simulink model "mce"  (Simulink 6.5)
settings: Solver=ode45  StartTime=0.0  StopTime=10.0  RelTol=1e-3
libraries: cdsFilt x334, cdsMatrix x9, cdsSwitch x7, cdsWD x7, cdsMuxMatrix x5, dac x3, cdsEpicsOut x2, cdsParameters x1
(part 10 of 18)

== system mce/Q1/M0/E/YAW ==
  In1 : Inport
  In2 : Inport  Port=2
  ADD : Subsystem
  CON : Subsystem
  SIG : Subsystem
  Out1 : Outport
  Out2 : Outport  Port=2
  Out3 : Outport  Port=3
  Out4 : Outport  Port=4
  wires:
  In1/1 -> SIG/1(In1)
  In2/1 -> CON/1(In1)
  SIG/1(Out1) -> ADD/1(In1)
  SIG/2(Out2) -> ADD/2(In2)
  SIG/3(Out3) -> ADD/3(In3)
  SIG/4(Out4) -> ADD/4(In4)
  CON/1(Out1) -> ADD/5(In17)
  CON/2(Out2) -> ADD/6(In18)
  CON/3(Out3) -> ADD/7(In19)
  CON/4(Out4) -> ADD/8(In20)
  ADD/1(Out1) -> Out1/1
  ADD/2(Out2) -> Out2/1
  ADD/3(Out3) -> Out3/1
  ADD/4(Out4) -> Out4/1

== system mce/Q1/M0/E/Z ==
  In1 : Inport
  In2 : Inport  Port=2
  ADD : Subsystem
  CON : Subsystem
  SIG : Subsystem
  Out1 : Outport
  Out2 : Outport  Port=2
  Out3 : Outport  Port=3
  Out4 : Outport  Port=4
  wires:
  In1/1 -> SIG/1(In1)
  In2/1 -> CON/1(In1)
  SIG/1(Out1) -> ADD/1(In1)
  SIG/2(Out2) -> ADD/2(In2)
  SIG/3(Out3) -> ADD/3(In3)
  SIG/4(Out4) -> ADD/4(In4)
  CON/1(Out1) -> ADD/5(In17)
  CON/2(Out2) -> ADD/6(In18)
  CON/3(Out3) -> ADD/7(In19)
  CON/4(Out4) -> ADD/8(In20)
  ADD/1(Out1) -> Out1/1
  ADD/2(Out2) -> Out2/1
  ADD/3(Out3) -> Out3/1
  ADD/4(Out4) -> Out4/1

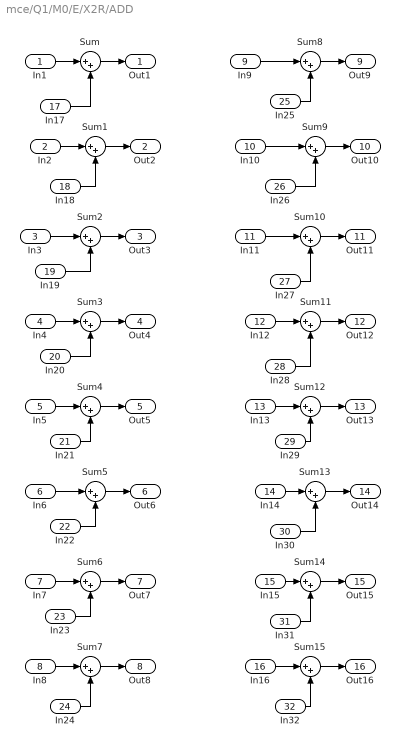
== system mce/Q1/M0/E/X2R/ADD ==
  In1 : Inport
  In2 : Inport  Port=2
  In3 : Inport  Port=3
  In4 : Inport  Port=4
  In5 : Inport  Port=5
  In6 : Inport  Port=6
  In7 : Inport  Port=7
  In8 : Inport  Port=8
  In9 : Inport  Port=9
  In10 : Inport  Port=10
  In11 : Inport  Port=11
  In12 : Inport  Port=12
  In13 : Inport  Port=13
  In14 : Inport  Port=14
  In15 : Inport  Port=15
  In16 : Inport  Port=16
  In17 : Inport  Port=17
  In18 : Inport  Port=18
  In19 : Inport  Port=19
  In20 : Inport  Port=20
  In21 : Inport  Port=21
  In22 : Inport  Port=22
  In23 : Inport  Port=23
  In24 : Inport  Port=24
  In25 : Inport  Port=25
  In26 : Inport  Port=26
  In27 : Inport  Port=27
  In28 : Inport  Port=28
  In29 : Inport  Port=29
  In30 : Inport  Port=30
  In31 : Inport  Port=31
  In32 : Inport  Port=32
  Sum{,1..15} (16 alike) : Sum  Inputs=|++
  Out1 : Outport
  Out2 : Outport  Port=2
  Out3 : Outport  Port=3
  Out4 : Outport  Port=4
  Out5 : Outport  Port=5
  Out6 : Outport  Port=6
  Out7 : Outport  Port=7
  Out8 : Outport  Port=8
  Out9 : Outport  Port=9
  Out10 : Outport  Port=10
  Out11 : Outport  Port=11
  Out12 : Outport  Port=12
  Out13 : Outport  Port=13
  Out14 : Outport  Port=14
  Out15 : Outport  Port=15
  Out16 : Outport  Port=16
  wires:
  In1/1 -> Sum/1
  Sum/1 -> Out1/1
  Sum1/1 -> Out2/1
  Sum2/1 -> Out3/1
  Sum3/1 -> Out4/1
  Sum4/1 -> Out5/1
  Sum5/1 -> Out6/1
  Sum6/1 -> Out7/1
  Sum7/1 -> Out8/1
  Sum8/1 -> Out9/1
  Sum9/1 -> Out10/1
  Sum10/1 -> Out11/1
  Sum11/1 -> Out12/1
  Sum12/1 -> Out13/1
  Sum13/1 -> Out14/1
  Sum14/1 -> Out15/1
  Sum15/1 -> Out16/1
  In17/1 -> Sum/2
  In2/1 -> Sum1/1
  In3/1 -> Sum2/1
  In4/1 -> Sum3/1
  In5/1 -> Sum4/1
  In19/1 -> Sum2/2
  In20/1 -> Sum3/2
  In21/1 -> Sum4/2
  In6/1 -> Sum5/1
  In22/1 -> Sum5/2
  In7/1 -> Sum6/1
  In23/1 -> Sum6/2
  In8/1 -> Sum7/1
  In24/1 -> Sum7/2
  In9/1 -> Sum8/1
  In25/1 -> Sum8/2
  In10/1 -> Sum9/1
  In26/1 -> Sum9/2
  In11/1 -> Sum10/1
  In27/1 -> Sum10/2
  In12/1 -> Sum11/1
  In28/1 -> Sum11/2
  In13/1 -> Sum12/1
  In29/1 -> Sum12/2
  In14/1 -> Sum13/1
  In30/1 -> Sum13/2
  In15/1 -> Sum14/1
  In31/1 -> Sum14/2
  In16/1 -> Sum15/1
  In32/1 -> Sum15/2
  In18/1 -> Sum1/2

== system mce/Q1/M0/E/X2R/CON ==
  In1 : Inport
  In2 : Inport  Port=2
  In3 : Inport  Port=3
  In4 : Inport  Port=4
  ADD : Subsystem
  ADD1 : Subsystem
  ADD3 : Subsystem
  P : Subsystem
  R : Subsystem
  X : Subsystem
  Y : Subsystem
  Out1 : Outport
  Out2 : Outport  Port=2
  Out3 : Outport  Port=3
  Out4 : Outport  Port=4
  Out5 : Outport  Port=5
  Out6 : Outport  Port=6
  Out7 : Outport  Port=7
  Out8 : Outport  Port=8
  Out9 : Outport  Port=9
  Out10 : Outport  Port=10
  Out11 : Outport  Port=11
  Out12 : Outport  Port=12
  Out13 : Outport  Port=13
  Out14 : Outport  Port=14
  Out15 : Outport  Port=15
  Out16 : Outport  Port=16
  wires:
  In1/1 -> X/1(In1)
  In2/1 -> Y/1(In1)
  X/1(Out1) -> ADD/1(In1)
  X/2(Out2) -> ADD/2(In2)
  X/3(Out3) -> ADD/3(In3)
  X/4(Out4) -> ADD/4(In4)
  X/5(Out5) -> ADD/5(In5)
  X/6(Out6) -> ADD/6(In6)
  X/7(Out7) -> ADD/7(In7)
  X/8(Out8) -> ADD/8(In8)
  X/9(Out9) -> ADD/9(In9)
  X/10(Out10) -> ADD/10(In10)
  X/11(Out11) -> ADD/11(In11)
  X/12(Out12) -> ADD/12(In12)
  X/13(Out13) -> ADD/13(In13)
  X/14(Out14) -> ADD/14(In14)
  X/15(Out15) -> ADD/15(In15)
  X/16(Out16) -> ADD/16(In16)
  In3/1 -> P/1(In1)
  In4/1 -> R/1(In1)
  ADD/1(Out1) -> ADD3/1(In1)
  ADD/2(Out2) -> ADD3/2(In2)
  ADD/3(Out3) -> ADD3/3(In3)
  ADD/4(Out4) -> ADD3/4(In4)
  ADD/5(Out5) -> ADD3/5(In5)
  ADD/6(Out6) -> ADD3/6(In6)
  ADD/7(Out7) -> ADD3/7(In7)
  ADD/8(Out8) -> ADD3/8(In8)
  ADD/9(Out9) -> ADD3/9(In9)
  ADD/10(Out10) -> ADD3/10(In10)
  ADD/11(Out11) -> ADD3/11(In11)
  ADD/12(Out12) -> ADD3/12(In12)
  ADD/13(Out13) -> ADD3/13(In13)
  ADD/14(Out14) -> ADD3/14(In14)
  ADD/15(Out15) -> ADD3/15(In15)
  ADD/16(Out16) -> ADD3/16(In16)
  ADD1/1(Out1) -> ADD3/17(In17)
  ADD1/2(Out2) -> ADD3/18(In18)
  ADD1/3(Out3) -> ADD3/19(In19)
  ADD1/4(Out4) -> ADD3/20(In20)
  ADD1/5(Out5) -> ADD3/21(In21)
  ADD1/6(Out6) -> ADD3/22(In22)
  ADD1/7(Out7) -> ADD3/23(In23)
  ADD1/8(Out8) -> ADD3/24(In24)
  ADD1/9(Out9) -> ADD3/25(In25)
  ADD1/10(Out10) -> ADD3/26(In26)
  ADD1/11(Out11) -> ADD3/27(In27)
  ADD1/12(Out12) -> ADD3/28(In28)
  ADD1/13(Out13) -> ADD3/29(In29)
  ADD1/14(Out14) -> ADD3/30(In30)
  ADD1/15(Out15) -> ADD3/31(In31)
  ADD1/16(Out16) -> ADD3/32(In32)
  ADD3/1(Out1) -> Out1/1
  ADD3/2(Out2) -> Out2/1
  ADD3/3(Out3) -> Out3/1
  ADD3/4(Out4) -> Out4/1
  ADD3/5(Out5) -> Out5/1
  ADD3/6(Out6) -> Out6/1
  ADD3/7(Out7) -> Out7/1
  ADD3/8(Out8) -> Out8/1
  ADD3/9(Out9) -> Out9/1
  ADD3/10(Out10) -> Out10/1
  ADD3/11(Out11) -> Out11/1
  ADD3/12(Out12) -> Out12/1
  ADD3/13(Out13) -> Out13/1
  ADD3/14(Out14) -> Out14/1
  ADD3/15(Out15) -> Out15/1
  ADD3/16(Out16) -> Out16/1
  Y/1(Out1) -> ADD/17(In17)
  Y/2(Out2) -> ADD/18(In18)
  Y/3(Out3) -> ADD/19(In19)
  Y/4(Out4) -> ADD/20(In20)
  Y/5(Out5) -> ADD/21(In21)
  Y/6(Out6) -> ADD/22(In22)
  Y/7(Out7) -> ADD/23(In23)
  Y/8(Out8) -> ADD/24(In24)
  Y/9(Out9) -> ADD/25(In25)
  Y/10(Out10) -> ADD/26(In26)
  Y/11(Out11) -> ADD/27(In27)
  Y/12(Out12) -> ADD/28(In28)
  Y/13(Out13) -> ADD/29(In29)
  Y/14(Out14) -> ADD/30(In30)
  Y/15(Out15) -> ADD/31(In31)
  Y/16(Out16) -> ADD/32(In32)
  P/1(Out1) -> ADD1/1(In1)
  P/2(Out2) -> ADD1/2(In2)
  P/3(Out3) -> ADD1/3(In3)
  P/4(Out4) -> ADD1/4(In4)
  P/5(Out5) -> ADD1/5(In5)
  P/6(Out6) -> ADD1/6(In6)
  P/7(Out7) -> ADD1/7(In7)
  P/8(Out8) -> ADD1/8(In8)
  P/9(Out9) -> ADD1/9(In9)
  P/10(Out10) -> ADD1/10(In10)
  P/11(Out11) -> ADD1/11(In11)
  P/12(Out12) -> ADD1/12(In12)
  P/13(Out13) -> ADD1/13(In13)
  P/14(Out14) -> ADD1/14(In14)
  P/15(Out15) -> ADD1/15(In15)
  P/16(Out16) -> ADD1/16(In16)
  R/1(Out1) -> ADD1/17(In17)
  R/2(Out2) -> ADD1/18(In18)
  R/3(Out3) -> ADD1/19(In19)
  R/4(Out4) -> ADD1/20(In20)
  R/5(Out5) -> ADD1/21(In21)
  R/6(Out6) -> ADD1/22(In22)
  R/7(Out7) -> ADD1/23(In23)
  R/8(Out8) -> ADD1/24(In24)
  R/9(Out9) -> ADD1/25(In25)
  R/10(Out10) -> ADD1/26(In26)
  R/11(Out11) -> ADD1/27(In27)
  R/12(Out12) -> ADD1/28(In28)
  R/13(Out13) -> ADD1/29(In29)
  R/14(Out14) -> ADD1/30(In30)
  R/15(Out15) -> ADD1/31(In31)
  R/16(Out16) -> ADD1/32(In32)

== system mce/Q1/M0/E/X2R/SIG ==
  In1 : Inport
  In2 : Inport  Port=2
  In3 : Inport  Port=3
  In4 : Inport  Port=4
  ADD : Subsystem
  ADD1 : Subsystem
  ADD3 : Subsystem
  P : Subsystem
  R : Subsystem
  X : Subsystem
  Y : Subsystem
  Out1 : Outport
  Out2 : Outport  Port=2
  Out3 : Outport  Port=3
  Out4 : Outport  Port=4
  Out5 : Outport  Port=5
  Out6 : Outport  Port=6
  Out7 : Outport  Port=7
  Out8 : Outport  Port=8
  Out9 : Outport  Port=9
  Out10 : Outport  Port=10
  Out11 : Outport  Port=11
  Out12 : Outport  Port=12
  Out13 : Outport  Port=13
  Out14 : Outport  Port=14
  Out15 : Outport  Port=15
  Out16 : Outport  Port=16
  wires:
  In1/1 -> X/1(In1)
  In2/1 -> Y/1(In1)
  X/1(Out1) -> ADD/1(In1)
  X/2(Out2) -> ADD/2(In2)
  X/3(Out3) -> ADD/3(In3)
  X/4(Out4) -> ADD/4(In4)
  X/5(Out5) -> ADD/5(In5)
  X/6(Out6) -> ADD/6(In6)
  X/7(Out7) -> ADD/7(In7)
  X/8(Out8) -> ADD/8(In8)
  X/9(Out9) -> ADD/9(In9)
  X/10(Out10) -> ADD/10(In10)
  X/11(Out11) -> ADD/11(In11)
  X/12(Out12) -> ADD/12(In12)
  X/13(Out13) -> ADD/13(In13)
  X/14(Out14) -> ADD/14(In14)
  X/15(Out15) -> ADD/15(In15)
  X/16(Out16) -> ADD/16(In16)
  In3/1 -> P/1(In1)
  In4/1 -> R/1(In1)
  ADD/1(Out1) -> ADD3/1(In1)
  ADD/2(Out2) -> ADD3/2(In2)
  ADD/3(Out3) -> ADD3/3(In3)
  ADD/4(Out4) -> ADD3/4(In4)
  ADD/5(Out5) -> ADD3/5(In5)
  ADD/6(Out6) -> ADD3/6(In6)
  ADD/7(Out7) -> ADD3/7(In7)
  ADD/8(Out8) -> ADD3/8(In8)
  ADD/9(Out9) -> ADD3/9(In9)
  ADD/10(Out10) -> ADD3/10(In10)
  ADD/11(Out11) -> ADD3/11(In11)
  ADD/12(Out12) -> ADD3/12(In12)
  ADD/13(Out13) -> ADD3/13(In13)
  ADD/14(Out14) -> ADD3/14(In14)
  ADD/15(Out15) -> ADD3/15(In15)
  ADD/16(Out16) -> ADD3/16(In16)
  ADD1/1(Out1) -> ADD3/17(In17)
  ADD1/2(Out2) -> ADD3/18(In18)
  ADD1/3(Out3) -> ADD3/19(In19)
  ADD1/4(Out4) -> ADD3/20(In20)
  ADD1/5(Out5) -> ADD3/21(In21)
  ADD1/6(Out6) -> ADD3/22(In22)
  ADD1/7(Out7) -> ADD3/23(In23)
  ADD1/8(Out8) -> ADD3/24(In24)
  ADD1/9(Out9) -> ADD3/25(In25)
  ADD1/10(Out10) -> ADD3/26(In26)
  ADD1/11(Out11) -> ADD3/27(In27)
  ADD1/12(Out12) -> ADD3/28(In28)
  ADD1/13(Out13) -> ADD3/29(In29)
  ADD1/14(Out14) -> ADD3/30(In30)
  ADD1/15(Out15) -> ADD3/31(In31)
  ADD1/16(Out16) -> ADD3/32(In32)
  ADD3/1(Out1) -> Out1/1
  ADD3/2(Out2) -> Out2/1
  ADD3/3(Out3) -> Out3/1
  ADD3/4(Out4) -> Out4/1
  ADD3/5(Out5) -> Out5/1
  ADD3/6(Out6) -> Out6/1
  ADD3/7(Out7) -> Out7/1
  ADD3/8(Out8) -> Out8/1
  ADD3/9(Out9) -> Out9/1
  ADD3/10(Out10) -> Out10/1
  ADD3/11(Out11) -> Out11/1
  ADD3/12(Out12) -> Out12/1
  ADD3/13(Out13) -> Out13/1
  ADD3/14(Out14) -> Out14/1
  ADD3/15(Out15) -> Out15/1
  ADD3/16(Out16) -> Out16/1
  Y/1(Out1) -> ADD/17(In17)
  Y/2(Out2) -> ADD/18(In18)
  Y/3(Out3) -> ADD/19(In19)
  Y/4(Out4) -> ADD/20(In20)
  Y/5(Out5) -> ADD/21(In21)
  Y/6(Out6) -> ADD/22(In22)
  Y/7(Out7) -> ADD/23(In23)
  Y/8(Out8) -> ADD/24(In24)
  Y/9(Out9) -> ADD/25(In25)
  Y/10(Out10) -> ADD/26(In26)
  Y/11(Out11) -> ADD/27(In27)
  Y/12(Out12) -> ADD/28(In28)
  Y/13(Out13) -> ADD/29(In29)
  Y/14(Out14) -> ADD/30(In30)
  Y/15(Out15) -> ADD/31(In31)
  Y/16(Out16) -> ADD/32(In32)
  P/1(Out1) -> ADD1/1(In1)
  P/2(Out2) -> ADD1/2(In2)
  P/3(Out3) -> ADD1/3(In3)
  P/4(Out4) -> ADD1/4(In4)
  P/5(Out5) -> ADD1/5(In5)
  P/6(Out6) -> ADD1/6(In6)
  P/7(Out7) -> ADD1/7(In7)
  P/8(Out8) -> ADD1/8(In8)
  P/9(Out9) -> ADD1/9(In9)
  P/10(Out10) -> ADD1/10(In10)
  P/11(Out11) -> ADD1/11(In11)
  P/12(Out12) -> ADD1/12(In12)
  P/13(Out13) -> ADD1/13(In13)
  P/14(Out14) -> ADD1/14(In14)
  P/15(Out15) -> ADD1/15(In15)
  P/16(Out16) -> ADD1/16(In16)
  R/1(Out1) -> ADD1/17(In17)
  R/2(Out2) -> ADD1/18(In18)
  R/3(Out3) -> ADD1/19(In19)
  R/4(Out4) -> ADD1/20(In20)
  R/5(Out5) -> ADD1/21(In21)
  R/6(Out6) -> ADD1/22(In22)
  R/7(Out7) -> ADD1/23(In23)
  R/8(Out8) -> ADD1/24(In24)
  R/9(Out9) -> ADD1/25(In25)
  R/10(Out10) -> ADD1/26(In26)
  R/11(Out11) -> ADD1/27(In27)
  R/12(Out12) -> ADD1/28(In28)
  R/13(Out13) -> ADD1/29(In29)
  R/14(Out14) -> ADD1/30(In30)
  R/15(Out15) -> ADD1/31(In31)
  R/16(Out16) -> ADD1/32(In32)

== system mce/Q1/M0/E/YAW/ADD ==
  In1 : Inport
  In2 : Inport  Port=2
  In3 : Inport  Port=3
  In4 : Inport  Port=4
  In17 : Inport  Port=5
  In18 : Inport  Port=6
  In19 : Inport  Port=7
  In20 : Inport  Port=8
  Sum{,1..3} (4 alike) : Sum  Inputs=|++
  Out1 : Outport
  Out2 : Outport  Port=2
  Out3 : Outport  Port=3
  Out4 : Outport  Port=4
  wires:
  In1/1 -> Sum/1
  Sum/1 -> Out1/1
  Sum1/1 -> Out2/1
  Sum2/1 -> Out3/1
  Sum3/1 -> Out4/1
  In17/1 -> Sum/2
  In2/1 -> Sum1/1
  In3/1 -> Sum2/1
  In4/1 -> Sum3/1
  In19/1 -> Sum2/2
  In20/1 -> Sum3/2
  In18/1 -> Sum1/2

== system mce/Q1/M0/E/YAW/CON ==
  In1 : Inport
  M1 : cdsFilt/Subsystem  Tag=cdsFilt  Description=|  SystemSampleTime=-1
      | Purpose:                                                                                                                                                                                                                                  
      | Standard CDS IIR filter module.                                                                                                                                                                                                           
      |                                                                                                                                                                                                                                           
      | Operation:                                                                                                                                                                                                                                
      | Consists of 10 second order section IIR filters, plus a ramped gain stage. In FE code, also provides pre-defined test points and excitation channel inputs. The filter coefficients are defined in the LIGO system using the 'foton' tool.
      |                                                                                                                                                                                                                                           
      | Usage:                                                                                                                                                                                                                                    
      | Name the part with the desired filter module name.
      settings: AttributesFormatString=%<Tag>
  M2 : cdsFilt/Subsystem  Tag=cdsFilt  Description=|  SystemSampleTime=-1
      | Purpose:                                                                                                                                                                                                                                  
      | Standard CDS IIR filter module.                                                                                                                                                                                                           
      |                                                                                                                                                                                                                                           
      | Operation:                                                                                                                                                                                                                                
      | Consists of 10 second order section IIR filters, plus a ramped gain stage. In FE code, also provides pre-defined test points and excitation channel inputs. The filter coefficients are defined in the LIGO system using the 'foton' tool.
      |                                                                                                                                                                                                                                           
      | Usage:                                                                                                                                                                                                                                    
      | Name the part with the desired filter module name.
      settings: AttributesFormatString=%<Tag>
  M3 : cdsFilt/Subsystem  Tag=cdsFilt  Description=|  SystemSampleTime=-1
      | Purpose:                                                                                                                                                                                                                                  
      | Standard CDS IIR filter module.                                                                                                                                                                                                           
      |                                                                                                                                                                                                                                           
      | Operation:                                                                                                                                                                                                                                
      | Consists of 10 second order section IIR filters, plus a ramped gain stage. In FE code, also provides pre-defined test points and excitation channel inputs. The filter coefficients are defined in the LIGO system using the 'foton' tool.
      |                                                                                                                                                                                                                                           
      | Usage:                                                                                                                                                                                                                                    
      | Name the part with the desired filter module name.
      settings: AttributesFormatString=%<Tag>
  M4 : cdsFilt/Subsystem  Tag=cdsFilt  Description=|  SystemSampleTime=-1
      | Purpose:                                                                                                                                                                                                                                  
      | Standard CDS IIR filter module.                                                                                                                                                                                                           
      |                                                                                                                                                                                                                                           
      | Operation:                                                                                                                                                                                                                                
      | Consists of 10 second order section IIR filters, plus a ramped gain stage. In FE code, also provides pre-defined test points and excitation channel inputs. The filter coefficients are defined in the LIGO system using the 'foton' tool.
      |                                                                                                                                                                                                                                           
      | Usage:                                                                                                                                                                                                                                    
      | Name the part with the desired filter module name.
      settings: AttributesFormatString=%<Tag>
  Out1 : Outport
  Out2 : Outport  Port=2
  Out3 : Outport  Port=3
  Out4 : Outport  Port=4
  wires:
  M1/1 -> Out1/1
  M2/1 -> Out2/1
  M3/1 -> Out3/1
  M4/1 -> Out4/1
  In1/1 -> M1/1, M2/1, M3/1, M4/1

== system mce/Q1/M0/E/YAW/SIG ==
  In1 : Inport
  M1 : cdsFilt/Subsystem  Tag=cdsFilt  Description=|  SystemSampleTime=-1
      | Purpose:                                                                                                                                                                                                                                  
      | Standard CDS IIR filter module.                                                                                                                                                                                                           
      |                                                                                                                                                                                                                                           
      | Operation:                                                                                                                                                                                                                                
      | Consists of 10 second order section IIR filters, plus a ramped gain stage. In FE code, also provides pre-defined test points and excitation channel inputs. The filter coefficients are defined in the LIGO system using the 'foton' tool.
      |                                                                                                                                                                                                                                           
      | Usage:                                                                                                                                                                                                                                    
      | Name the part with the desired filter module name.
      settings: AttributesFormatString=%<Tag>
  M2 : cdsFilt/Subsystem  Tag=cdsFilt  Description=|  SystemSampleTime=-1
      | Purpose:                                                                                                                                                                                                                                  
      | Standard CDS IIR filter module.                                                                                                                                                                                                           
      |                                                                                                                                                                                                                                           
      | Operation:                                                                                                                                                                                                                                
      | Consists of 10 second order section IIR filters, plus a ramped gain stage. In FE code, also provides pre-defined test points and excitation channel inputs. The filter coefficients are defined in the LIGO system using the 'foton' tool.
      |                                                                                                                                                                                                                                           
      | Usage:                                                                                                                                                                                                                                    
      | Name the part with the desired filter module name.
      settings: AttributesFormatString=%<Tag>
  M3 : cdsFilt/Subsystem  Tag=cdsFilt  Description=|  SystemSampleTime=-1
      | Purpose:                                                                                                                                                                                                                                  
      | Standard CDS IIR filter module.                                                                                                                                                                                                           
      |                                                                                                                                                                                                                                           
      | Operation:                                                                                                                                                                                                                                
      | Consists of 10 second order section IIR filters, plus a ramped gain stage. In FE code, also provides pre-defined test points and excitation channel inputs. The filter coefficients are defined in the LIGO system using the 'foton' tool.
      |                                                                                                                                                                                                                                           
      | Usage:                                                                                                                                                                                                                                    
      | Name the part with the desired filter module name.
      settings: AttributesFormatString=%<Tag>
  M4 : cdsFilt/Subsystem  Tag=cdsFilt  Description=|  SystemSampleTime=-1
      | Purpose:                                                                                                                                                                                                                                  
      | Standard CDS IIR filter module.                                                                                                                                                                                                           
      |                                                                                                                                                                                                                                           
      | Operation:                                                                                                                                                                                                                                
      | Consists of 10 second order section IIR filters, plus a ramped gain stage. In FE code, also provides pre-defined test points and excitation channel inputs. The filter coefficients are defined in the LIGO system using the 'foton' tool.
      |                                                                                                                                                                                                                                           
      | Usage:                                                                                                                                                                                                                                    
      | Name the part with the desired filter module name.
      settings: AttributesFormatString=%<Tag>
  Out1 : Outport
  Out2 : Outport  Port=2
  Out3 : Outport  Port=3
  Out4 : Outport  Port=4
  wires:
  M1/1 -> Out1/1
  M2/1 -> Out2/1
  M3/1 -> Out3/1
  M4/1 -> Out4/1
  In1/1 -> M2/1, M3/1, M4/1, M1/1

== system mce/Q1/M0/E/Z/ADD ==
  In1 : Inport
  In2 : Inport  Port=2
  In3 : Inport  Port=3
  In4 : Inport  Port=4
  In17 : Inport  Port=5
  In18 : Inport  Port=6
  In19 : Inport  Port=7
  In20 : Inport  Port=8
  Sum{,1..3} (4 alike) : Sum  Inputs=|++
  Out1 : Outport
  Out2 : Outport  Port=2
  Out3 : Outport  Port=3
  Out4 : Outport  Port=4
  wires:
  In1/1 -> Sum/1
  Sum/1 -> Out1/1
  Sum1/1 -> Out2/1
  Sum2/1 -> Out3/1
  Sum3/1 -> Out4/1
  In17/1 -> Sum/2
  In2/1 -> Sum1/1
  In3/1 -> Sum2/1
  In4/1 -> Sum3/1
  In19/1 -> Sum2/2
  In20/1 -> Sum3/2
  In18/1 -> Sum1/2

== system mce/Q1/M0/E/Z/CON ==
  In1 : Inport
  M1 : cdsFilt/Subsystem  Tag=cdsFilt  Description=|  SystemSampleTime=-1
      | Purpose:                                                                                                                                                                                                                                  
      | Standard CDS IIR filter module.                                                                                                                                                                                                           
      |                                                                                                                                                                                                                                           
      | Operation:                                                                                                                                                                                                                                
      | Consists of 10 second order section IIR filters, plus a ramped gain stage. In FE code, also provides pre-defined test points and excitation channel inputs. The filter coefficients are defined in the LIGO system using the 'foton' tool.
      |                                                                                                                                                                                                                                           
      | Usage:                                                                                                                                                                                                                                    
      | Name the part with the desired filter module name.
      settings: AttributesFormatString=%<Tag>
  M2 : cdsFilt/Subsystem  Tag=cdsFilt  Description=|  SystemSampleTime=-1
      | Purpose:                                                                                                                                                                                                                                  
      | Standard CDS IIR filter module.                                                                                                                                                                                                           
      |                                                                                                                                                                                                                                           
      | Operation:                                                                                                                                                                                                                                
      | Consists of 10 second order section IIR filters, plus a ramped gain stage. In FE code, also provides pre-defined test points and excitation channel inputs. The filter coefficients are defined in the LIGO system using the 'foton' tool.
      |                                                                                                                                                                                                                                           
      | Usage:                                                                                                                                                                                                                                    
      | Name the part with the desired filter module name.
      settings: AttributesFormatString=%<Tag>
  M3 : cdsFilt/Subsystem  Tag=cdsFilt  Description=|  SystemSampleTime=-1
      | Purpose:                                                                                                                                                                                                                                  
      | Standard CDS IIR filter module.                                                                                                                                                                                                           
      |                                                                                                                                                                                                                                           
      | Operation:                                                                                                                                                                                                                                
      | Consists of 10 second order section IIR filters, plus a ramped gain stage. In FE code, also provides pre-defined test points and excitation channel inputs. The filter coefficients are defined in the LIGO system using the 'foton' tool.
      |                                                                                                                                                                                                                                           
      | Usage:                                                                                                                                                                                                                                    
      | Name the part with the desired filter module name.
      settings: AttributesFormatString=%<Tag>
  M4 : cdsFilt/Subsystem  Tag=cdsFilt  Description=|  SystemSampleTime=-1
      | Purpose:                                                                                                                                                                                                                                  
      | Standard CDS IIR filter module.                                                                                                                                                                                                           
      |                                                                                                                                                                                                                                           
      | Operation:                                                                                                                                                                                                                                
      | Consists of 10 second order section IIR filters, plus a ramped gain stage. In FE code, also provides pre-defined test points and excitation channel inputs. The filter coefficients are defined in the LIGO system using the 'foton' tool.
      |                                                                                                                                                                                                                                           
      | Usage:                                                                                                                                                                                                                                    
      | Name the part with the desired filter module name.
      settings: AttributesFormatString=%<Tag>
  Out1 : Outport
  Out2 : Outport  Port=2
  Out3 : Outport  Port=3
  Out4 : Outport  Port=4
  wires:
  M1/1 -> Out1/1
  M2/1 -> Out2/1
  M3/1 -> Out3/1
  M4/1 -> Out4/1
  In1/1 -> M1/1, M2/1, M3/1, M4/1

== system mce/Q1/M0/E/Z/SIG ==
  In1 : Inport
  M1 : cdsFilt/Subsystem  Tag=cdsFilt  Description=|  SystemSampleTime=-1
      | Purpose:                                                                                                                                                                                                                                  
      | Standard CDS IIR filter module.                                                                                                                                                                                                           
      |                                                                                                                                                                                                                                           
      | Operation:                                                                                                                                                                                                                                
      | Consists of 10 second order section IIR filters, plus a ramped gain stage. In FE code, also provides pre-defined test points and excitation channel inputs. The filter coefficients are defined in the LIGO system using the 'foton' tool.
      |                                                                                                                                                                                                                                           
      | Usage:                                                                                                                                                                                                                                    
      | Name the part with the desired filter module name.
      settings: AttributesFormatString=%<Tag>
  M2 : cdsFilt/Subsystem  Tag=cdsFilt  Description=|  SystemSampleTime=-1
      | Purpose:                                                                                                                                                                                                                                  
      | Standard CDS IIR filter module.                                                                                                                                                                                                           
      |                                                                                                                                                                                                                                           
      | Operation:                                                                                                                                                                                                                                
      | Consists of 10 second order section IIR filters, plus a ramped gain stage. In FE code, also provides pre-defined test points and excitation channel inputs. The filter coefficients are defined in the LIGO system using the 'foton' tool.
      |                                                                                                                                                                                                                                           
      | Usage:                                                                                                                                                                                                                                    
      | Name the part with the desired filter module name.
      settings: AttributesFormatString=%<Tag>
  M3 : cdsFilt/Subsystem  Tag=cdsFilt  Description=|  SystemSampleTime=-1
      | Purpose:                                                                                                                                                                                                                                  
      | Standard CDS IIR filter module.                                                                                                                                                                                                           
      |                                                                                                                                                                                                                                           
      | Operation:                                                                                                                                                                                                                                
      | Consists of 10 second order section IIR filters, plus a ramped gain stage. In FE code, also provides pre-defined test points and excitation channel inputs. The filter coefficients are defined in the LIGO system using the 'foton' tool.
      |                                                                                                                                                                                                                                           
      | Usage:                                                                                                                                                                                                                                    
      | Name the part with the desired filter module name.
      settings: AttributesFormatString=%<Tag>
  M4 : cdsFilt/Subsystem  Tag=cdsFilt  Description=|  SystemSampleTime=-1
      | Purpose:                                                                                                                                                                                                                                  
      | Standard CDS IIR filter module.                                                                                                                                                                                                           
      |                                                                                                                                                                                                                                           
      | Operation:                                                                                                                                                                                                                                
      | Consists of 10 second order section IIR filters, plus a ramped gain stage. In FE code, also provides pre-defined test points and excitation channel inputs. The filter coefficients are defined in the LIGO system using the 'foton' tool.
      |                                                                                                                                                                                                                                           
      | Usage:                                                                                                                                                                                                                                    
      | Name the part with the desired filter module name.
      settings: AttributesFormatString=%<Tag>
  Out1 : Outport
  Out2 : Outport  Port=2
  Out3 : Outport  Port=3
  Out4 : Outport  Port=4
  wires:
  M1/1 -> Out1/1
  M2/1 -> Out2/1
  M3/1 -> Out3/1
  M4/1 -> Out4/1
  In1/1 -> M2/1, M3/1, M4/1, M1/1

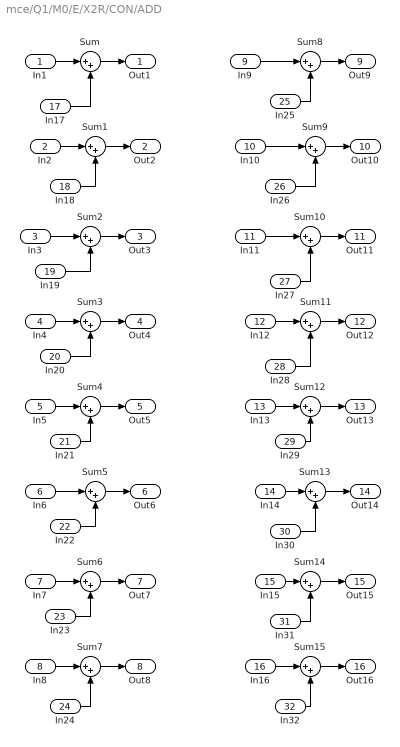
== system mce/Q1/M0/E/X2R/CON/ADD ==
  In1 : Inport
  In2 : Inport  Port=2
  In3 : Inport  Port=3
  In4 : Inport  Port=4
  In5 : Inport  Port=5
  In6 : Inport  Port=6
  In7 : Inport  Port=7
  In8 : Inport  Port=8
  In9 : Inport  Port=9
  In10 : Inport  Port=10
  In11 : Inport  Port=11
  In12 : Inport  Port=12
  In13 : Inport  Port=13
  In14 : Inport  Port=14
  In15 : Inport  Port=15
  In16 : Inport  Port=16
  In17 : Inport  Port=17
  In18 : Inport  Port=18
  In19 : Inport  Port=19
  In20 : Inport  Port=20
  In21 : Inport  Port=21
  In22 : Inport  Port=22
  In23 : Inport  Port=23
  In24 : Inport  Port=24
  In25 : Inport  Port=25
  In26 : Inport  Port=26
  In27 : Inport  Port=27
  In28 : Inport  Port=28
  In29 : Inport  Port=29
  In30 : Inport  Port=30
  In31 : Inport  Port=31
  In32 : Inport  Port=32
  Sum{,1..15} (16 alike) : Sum  Inputs=|++
  Out1 : Outport
  Out2 : Outport  Port=2
  Out3 : Outport  Port=3
  Out4 : Outport  Port=4
  Out5 : Outport  Port=5
  Out6 : Outport  Port=6
  Out7 : Outport  Port=7
  Out8 : Outport  Port=8
  Out9 : Outport  Port=9
  Out10 : Outport  Port=10
  Out11 : Outport  Port=11
  Out12 : Outport  Port=12
  Out13 : Outport  Port=13
  Out14 : Outport  Port=14
  Out15 : Outport  Port=15
  Out16 : Outport  Port=16
  wires:
  In1/1 -> Sum/1
  Sum/1 -> Out1/1
  Sum1/1 -> Out2/1
  Sum2/1 -> Out3/1
  Sum3/1 -> Out4/1
  Sum4/1 -> Out5/1
  Sum5/1 -> Out6/1
  Sum6/1 -> Out7/1
  Sum7/1 -> Out8/1
  Sum8/1 -> Out9/1
  Sum9/1 -> Out10/1
  Sum10/1 -> Out11/1
  Sum11/1 -> Out12/1
  Sum12/1 -> Out13/1
  Sum13/1 -> Out14/1
  Sum14/1 -> Out15/1
  Sum15/1 -> Out16/1
  In17/1 -> Sum/2
  In2/1 -> Sum1/1
  In3/1 -> Sum2/1
  In4/1 -> Sum3/1
  In5/1 -> Sum4/1
  In19/1 -> Sum2/2
  In20/1 -> Sum3/2
  In21/1 -> Sum4/2
  In6/1 -> Sum5/1
  In22/1 -> Sum5/2
  In7/1 -> Sum6/1
  In23/1 -> Sum6/2
  In8/1 -> Sum7/1
  In24/1 -> Sum7/2
  In9/1 -> Sum8/1
  In25/1 -> Sum8/2
  In10/1 -> Sum9/1
  In26/1 -> Sum9/2
  In11/1 -> Sum10/1
  In27/1 -> Sum10/2
  In12/1 -> Sum11/1
  In28/1 -> Sum11/2
  In13/1 -> Sum12/1
  In29/1 -> Sum12/2
  In14/1 -> Sum13/1
  In30/1 -> Sum13/2
  In15/1 -> Sum14/1
  In31/1 -> Sum14/2
  In16/1 -> Sum15/1
  In32/1 -> Sum15/2
  In18/1 -> Sum1/2

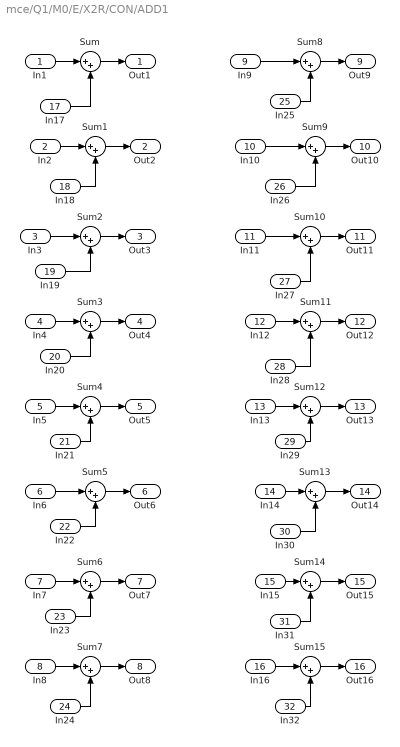
== system mce/Q1/M0/E/X2R/CON/ADD1 ==
  In1 : Inport
  In2 : Inport  Port=2
  In3 : Inport  Port=3
  In4 : Inport  Port=4
  In5 : Inport  Port=5
  In6 : Inport  Port=6
  In7 : Inport  Port=7
  In8 : Inport  Port=8
  In9 : Inport  Port=9
  In10 : Inport  Port=10
  In11 : Inport  Port=11
  In12 : Inport  Port=12
  In13 : Inport  Port=13
  In14 : Inport  Port=14
  In15 : Inport  Port=15
  In16 : Inport  Port=16
  In17 : Inport  Port=17
  In18 : Inport  Port=18
  In19 : Inport  Port=19
  In20 : Inport  Port=20
  In21 : Inport  Port=21
  In22 : Inport  Port=22
  In23 : Inport  Port=23
  In24 : Inport  Port=24
  In25 : Inport  Port=25
  In26 : Inport  Port=26
  In27 : Inport  Port=27
  In28 : Inport  Port=28
  In29 : Inport  Port=29
  In30 : Inport  Port=30
  In31 : Inport  Port=31
  In32 : Inport  Port=32
  Sum{,1..15} (16 alike) : Sum  Inputs=|++
  Out1 : Outport
  Out2 : Outport  Port=2
  Out3 : Outport  Port=3
  Out4 : Outport  Port=4
  Out5 : Outport  Port=5
  Out6 : Outport  Port=6
  Out7 : Outport  Port=7
  Out8 : Outport  Port=8
  Out9 : Outport  Port=9
  Out10 : Outport  Port=10
  Out11 : Outport  Port=11
  Out12 : Outport  Port=12
  Out13 : Outport  Port=13
  Out14 : Outport  Port=14
  Out15 : Outport  Port=15
  Out16 : Outport  Port=16
  wires:
  In1/1 -> Sum/1
  Sum/1 -> Out1/1
  Sum1/1 -> Out2/1
  Sum2/1 -> Out3/1
  Sum3/1 -> Out4/1
  Sum4/1 -> Out5/1
  Sum5/1 -> Out6/1
  Sum6/1 -> Out7/1
  Sum7/1 -> Out8/1
  Sum8/1 -> Out9/1
  Sum9/1 -> Out10/1
  Sum10/1 -> Out11/1
  Sum11/1 -> Out12/1
  Sum12/1 -> Out13/1
  Sum13/1 -> Out14/1
  Sum14/1 -> Out15/1
  Sum15/1 -> Out16/1
  In17/1 -> Sum/2
  In2/1 -> Sum1/1
  In3/1 -> Sum2/1
  In4/1 -> Sum3/1
  In5/1 -> Sum4/1
  In19/1 -> Sum2/2
  In20/1 -> Sum3/2
  In21/1 -> Sum4/2
  In6/1 -> Sum5/1
  In22/1 -> Sum5/2
  In7/1 -> Sum6/1
  In23/1 -> Sum6/2
  In8/1 -> Sum7/1
  In24/1 -> Sum7/2
  In9/1 -> Sum8/1
  In25/1 -> Sum8/2
  In10/1 -> Sum9/1
  In26/1 -> Sum9/2
  In11/1 -> Sum10/1
  In27/1 -> Sum10/2
  In12/1 -> Sum11/1
  In28/1 -> Sum11/2
  In13/1 -> Sum12/1
  In29/1 -> Sum12/2
  In14/1 -> Sum13/1
  In30/1 -> Sum13/2
  In15/1 -> Sum14/1
  In31/1 -> Sum14/2
  In16/1 -> Sum15/1
  In32/1 -> Sum15/2
  In18/1 -> Sum1/2
